simulink model "Inverse_dynamic_Cartesian_aJacobian"  (R2020b)
settings: Solver=VariableStepAuto  StartTime=0.0  StopTime=10.0  RelTol=1e-3
(part 1 of 5)
settings Model: Creator=Asus  LastModifiedBy=Asus

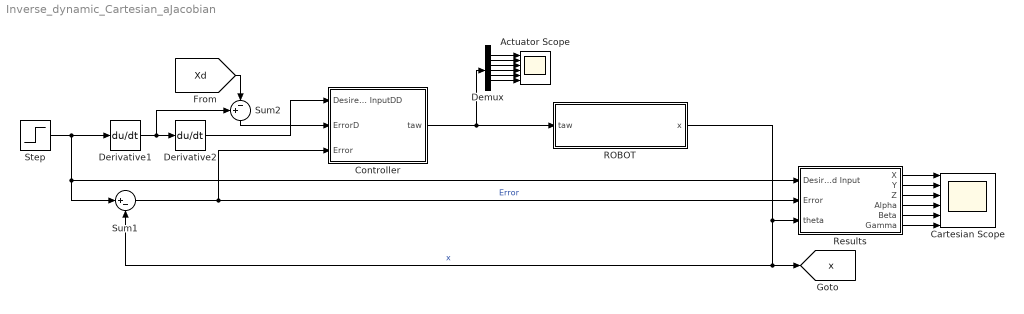
== system Inverse_dynamic_Cartesian_aJacobian ==
  Actuator Scope : Scope  NumInputPorts=6
  Cartesian Scope : Scope  NumInputPorts=6
  Controller : Subsystem
  Demux : Demux  Outputs=6
  Derivative1 : Derivative
  Derivative2 : Derivative
  ROBOT : Subsystem
  Results : Subsystem
  Step : Step  Time=0  Before=[0.5;0.5;1;pi/4;pi/2;pi/4];  After=[0.6;0.6;1.5;pi/6;pi/4;pi/3];  SampleTime=0
  Sum1 : Sum  Inputs=|+-
  Sum2 : Sum  Inputs=+-|
  tag scope: x=global
  wires:
  Results/3(Z) -> Cartesian Scope/3
  Derivative1/1 -> Sum2/1, Derivative2/1
  Demux/6 -> Actuator Scope/6
  Sum2/1 -> Controller/2(ErrorD)
  ROBOT/1(x) -> [x], Sum1/2, Results/3(theta)  "x"
  Results/4(Alpha) -> Cartesian Scope/4
  Derivative2/1 -> Controller/1(Desired InputDD)
  Controller/1(taw) -> ROBOT/1(taw), Demux/1
  Demux/2 -> Actuator Scope/2
  Demux/4 -> Actuator Scope/4
  Demux/5 -> Actuator Scope/5
  Results/5(Beta) -> Cartesian Scope/5
  Sum1/1 -> Results/2(Error), Controller/3(Error)  "Error"
  Demux/1 -> Actuator Scope/1
  [Xd] -> Sum2/2
  Results/1(X) -> Cartesian Scope/1
  Results/6(Gamma) -> Cartesian Scope/6
  Results/2(Y) -> Cartesian Scope/2
  Step/1 -> Sum1/1, Results/1(Desired Input), Derivative1/1
  Demux/3 -> Actuator Scope/3

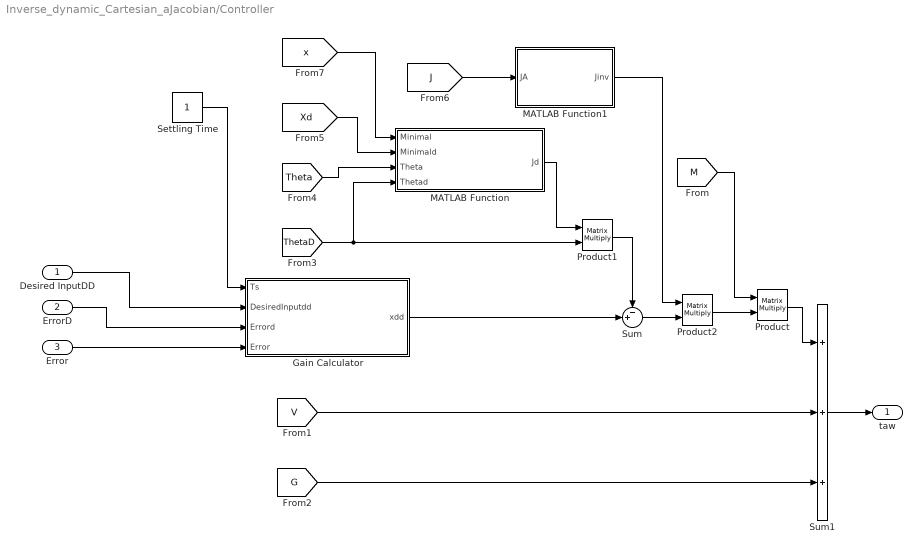
== system Inverse_dynamic_Cartesian_aJacobian/Controller ==
  Desired InputDD : Inport
  ErrorD : Inport  Port=2
  Error : Inport  Port=3
  Gain Calculator : MATLAB Function  TreatAsAtomicUnit=on
  MATLAB Function : MATLAB Function  TreatAsAtomicUnit=on
  MATLAB Function1 : MATLAB Function  TreatAsAtomicUnit=on
  Product : Product  Multiplication=Matrix(*)
  Product1 : Product  Multiplication=Matrix(*)
  Product2 : Product  Multiplication=Matrix(*)
  Settling Time : Constant
  Sum : Sum  Inputs=-+|
  Sum1 : Sum  Inputs=+++
  taw : Outport  VectorParamsAs1DForOutWhenUnconnected=off
  wires:
  [M] -> Product/1
  Gain Calculator/1(xdd) -> Sum/2
  Product/1 -> Sum1/1
  [V] -> Sum1/2
  [G] -> Sum1/3
  Settling Time/1 -> Gain Calculator/1(Ts)
  ErrorD/1 -> Gain Calculator/3(Errord)
  Error/1 -> Gain Calculator/4(Error)
  Desired InputDD/1 -> Gain Calculator/2(DesiredInputdd)
  Sum1/1 -> taw/1
  [ThetaD] -> MATLAB Function/4(Thetad), Product1/2
  Product1/1 -> Sum/1
  MATLAB Function/1(Jd) -> Product1/1
  Sum/1 -> Product2/2
  MATLAB Function1/1(Jinv) -> Product2/1
  Product2/1 -> Product/2
  [Theta] -> MATLAB Function/3(Theta)
  [J] -> MATLAB Function1/1(JA)
  [Xd] -> MATLAB Function/2(Minimald)
  [x] -> MATLAB Function/1(Minimal)

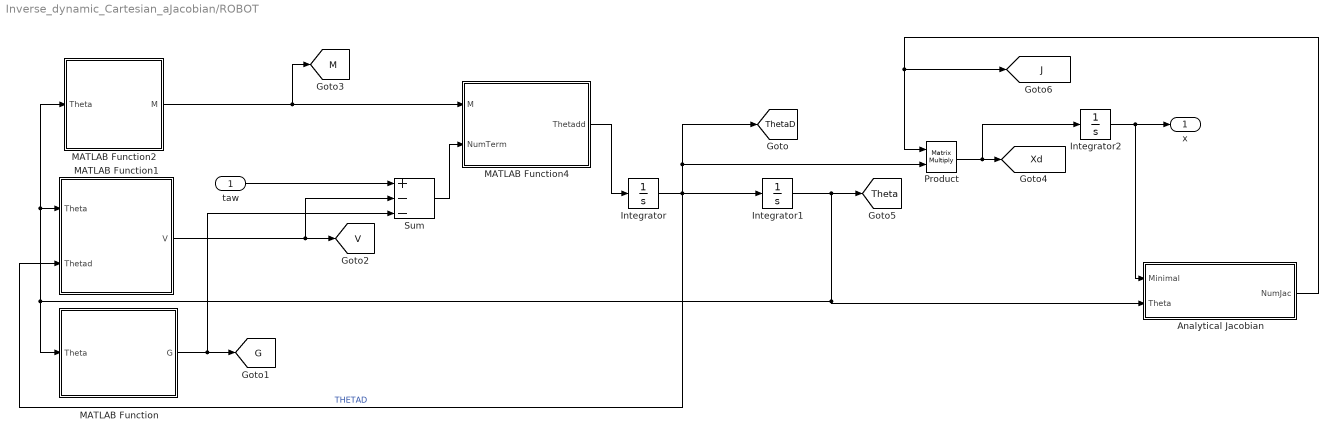
== system Inverse_dynamic_Cartesian_aJacobian/ROBOT ==
  taw : Inport
  Analytical Jacobian : MATLAB Function  TreatAsAtomicUnit=on
  Integrator : Integrator  InitialCondition=[0;0;0;0;0;0]
  Integrator1 : Integrator  InitialCondition=[0.659733742734682;-0.837199398722719;1.88109465000067;2.99646726889027;1.04847657950238;0.858183852099329];
  Integrator2 : Integrator  InitialCondition=[1.5;1.2;0.7;pi/4;pi/2;pi/4];
  MATLAB Function : MATLAB Function  TreatAsAtomicUnit=on
  MATLAB Function1 : MATLAB Function  TreatAsAtomicUnit=on
  MATLAB Function2 : MATLAB Function  TreatAsAtomicUnit=on
  MATLAB Function4 : MATLAB Function  TreatAsAtomicUnit=on
  Product : Product  Multiplication=Matrix(*)
  Sum : Sum  Inputs=+--
  x : Outport  VectorParamsAs1DForOutWhenUnconnected=off
  tag scope: G=global, J=global, M=global, Theta=global, ThetaD=global, V=global, Xd=global
  wires:
  Integrator1/1 -> MATLAB Function1/1(Theta), MATLAB Function2/1(Theta), MATLAB Function/1(Theta), Analytical Jacobian/2(Theta), [Theta]
  Product/1 -> Integrator2/1, [Xd]
  Integrator2/1 -> Analytical Jacobian/1(Minimal), x/1
  Analytical Jacobian/1(NumJac) -> Product/1, [J]
  MATLAB Function/1(G) -> [G], Sum/3
  MATLAB Function4/1(Thetadd) -> Integrator/1
  Sum/1 -> MATLAB Function4/2(NumTerm)
  taw/1 -> Sum/1
  MATLAB Function2/1(M) -> MATLAB Function4/1(M), [M]
  Integrator/1 -> Product/2, [ThetaD], MATLAB Function1/2(Thetad), Integrator1/1  "THETAD"
  MATLAB Function1/1(V) -> Sum/2, [V]

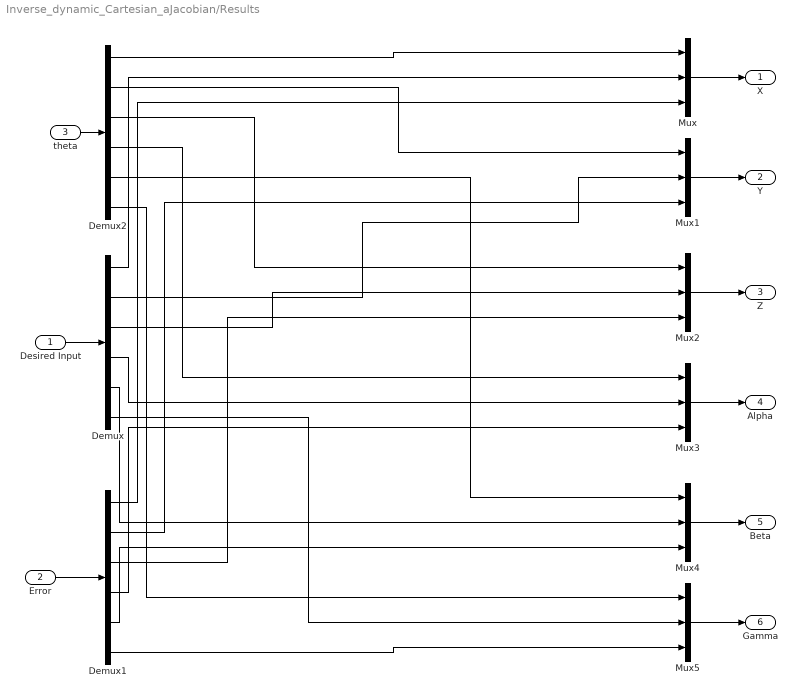
== system Inverse_dynamic_Cartesian_aJacobian/Results ==
  Desired Input : Inport
  Error : Inport  Port=2
  theta : Inport  Port=3
  Demux : Demux  Outputs=6
  Demux1 : Demux  Outputs=6
  Demux2 : Demux  Outputs=6
  Mux{,1..5} (6 alike) : Mux  Inputs=3
  X : Outport  VectorParamsAs1DForOutWhenUnconnected=off
  Y : Outport  Port=2  VectorParamsAs1DForOutWhenUnconnected=off
  Z : Outport  Port=3  VectorParamsAs1DForOutWhenUnconnected=off
  Alpha : Outport  Port=4  VectorParamsAs1DForOutWhenUnconnected=off
  Beta : Outport  Port=5  VectorParamsAs1DForOutWhenUnconnected=off
  Gamma : Outport  Port=6  VectorParamsAs1DForOutWhenUnconnected=off
  wires:
  Desired Input/1 -> Demux/1
  Error/1 -> Demux1/1
  theta/1 -> Demux2/1
  Mux/1 -> X/1
  Mux1/1 -> Y/1
  Mux2/1 -> Z/1
  Mux3/1 -> Alpha/1
  Mux4/1 -> Beta/1
  Mux5/1 -> Gamma/1
  Demux2/1 -> Mux/1
  Demux2/2 -> Mux1/1
  Demux2/3 -> Mux2/1
  Demux2/4 -> Mux3/1
  Demux2/5 -> Mux4/1
  Demux2/6 -> Mux5/1
  Demux/1 -> Mux/2
  Demux/2 -> Mux1/2
  Demux/3 -> Mux2/2
  Demux/4 -> Mux3/2
  Demux/5 -> Mux4/2
  Demux/6 -> Mux5/2
  Demux1/1 -> Mux/3
  Demux1/2 -> Mux1/3
  Demux1/3 -> Mux2/3
  Demux1/4 -> Mux3/3
  Demux1/5 -> Mux4/3
  Demux1/6 -> Mux5/3
